simulink model "prac5"  (R2019b)
settings: Solver=VariableStepAuto  StartTime=0.0  StopTime=10  RelTol=1e-3
values from neighbouring files (symbols this model uses):
  C = 0.97    [prac5_var.m]
  Td = 0.14    [prac5_var.m]
  wn = 4.75    [prac5_var.m]
  zw2 = 2*zeta*wn    (= 0.7695)    [prac5_var.m]
undefined symbols (not defined in the file or in its folder): a1, a2, a5, a6, cputime, den, num, num1, num2
settings Model: Creator=mluser  LastModifiedBy=waltd

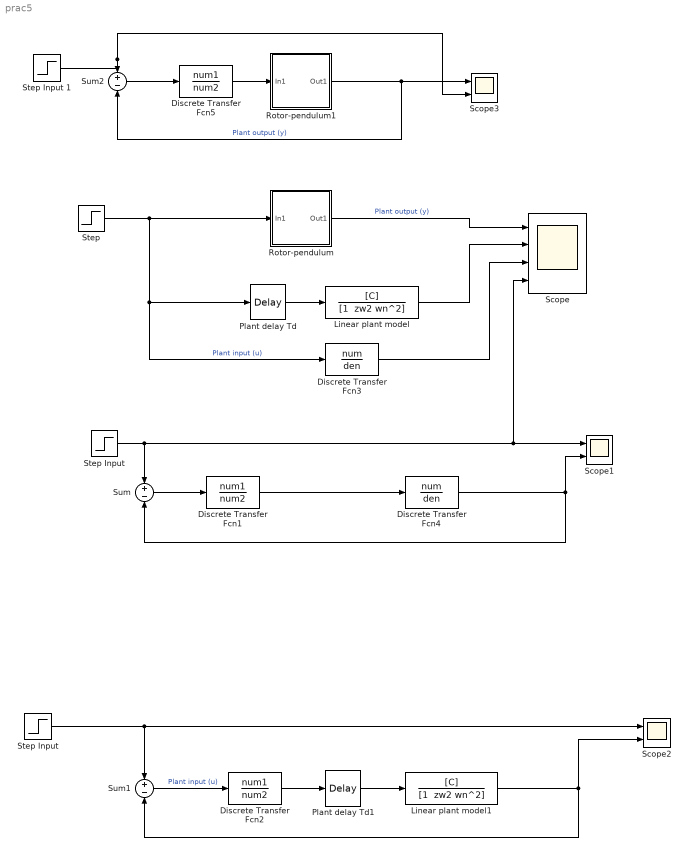
== system prac5 ==
  Discrete Transfer Fcn1 : DiscreteTransferFcn  Numerator=num1  Denominator=num2  SampleTime=0.15
  Discrete Transfer Fcn2 : DiscreteTransferFcn  Numerator=num1  Denominator=num2  SampleTime=0.15
  Discrete Transfer Fcn3 : DiscreteTransferFcn  Numerator=num  Denominator=den  SampleTime=0.15
  Discrete Transfer Fcn4 : DiscreteTransferFcn  Numerator=num  Denominator=den  SampleTime=0.15
  Discrete Transfer Fcn5 : DiscreteTransferFcn  Numerator=num1  Denominator=num2  SampleTime=0.15
  Linear plant model : TransferFcn  Numerator=[C]  Denominator="[1  zw2 wn^2]"
  Linear plant model1 : TransferFcn  Numerator=[C]  Denominator="[1  zw2 wn^2]"
  Plant delay Td : TransportDelay  DelayTime=Td
  Plant delay Td1 : TransportDelay  DelayTime=Td
  Rotor-pendulum : Subsystem  Description=Rotor pendulum
  Rotor-pendulum1 : Subsystem  Description=Rotor pendulum
  Scope : Scope  NumInputPorts=4
  Scope1 : Scope  NumInputPorts=2
  Scope2 : Scope  NumInputPorts=2
  Scope3 : Scope  NumInputPorts=2
  Step : Step  After=10  SampleTime=0
  "Step Input " : Step  After=0.5  SampleTime=0
  Step Input 1 : Step  After=0.5  SampleTime=0
  "Step Input " : Step  After=0.5  SampleTime=0
  Sum : Sum  Inputs=+-
  Sum1 : Sum  Inputs=+-
  Sum2 : Sum  Inputs=+-
  wires:
  Step/1 -> Rotor-pendulum/1(In1), Discrete Transfer Fcn3/1, Plant delay Td/1  "Plant input (u)"
  Rotor-pendulum/1(Out1) -> Scope/1  "Plant output (y)"
  Plant delay Td/1 -> Linear plant model/1
  Linear plant model/1 -> Scope/2
  Discrete Transfer Fcn1/1 -> Discrete Transfer Fcn4/1
  "Step Input "/1 -> Scope1/1, Scope/4, Sum/1
  Sum/1 -> Discrete Transfer Fcn1/1
  Plant delay Td1/1 -> Linear plant model1/1
  Sum1/1 -> Discrete Transfer Fcn2/1  "Plant input (u)"
  Linear plant model1/1 -> Scope2/2, Sum1/2
  Discrete Transfer Fcn2/1 -> Plant delay Td1/1
  "Step Input "/1 -> Scope2/1, Sum1/1
  Discrete Transfer Fcn3/1 -> Scope/3
  Discrete Transfer Fcn4/1 -> Scope1/2, Sum/2
  Discrete Transfer Fcn5/1 -> Rotor-pendulum1/1(In1)
  Rotor-pendulum1/1(Out1) -> Sum2/2, Scope3/1  "Plant output (y)"
  Step Input 1/1 -> Scope3/2, Sum2/1
  Sum2/1 -> Discrete Transfer Fcn5/1

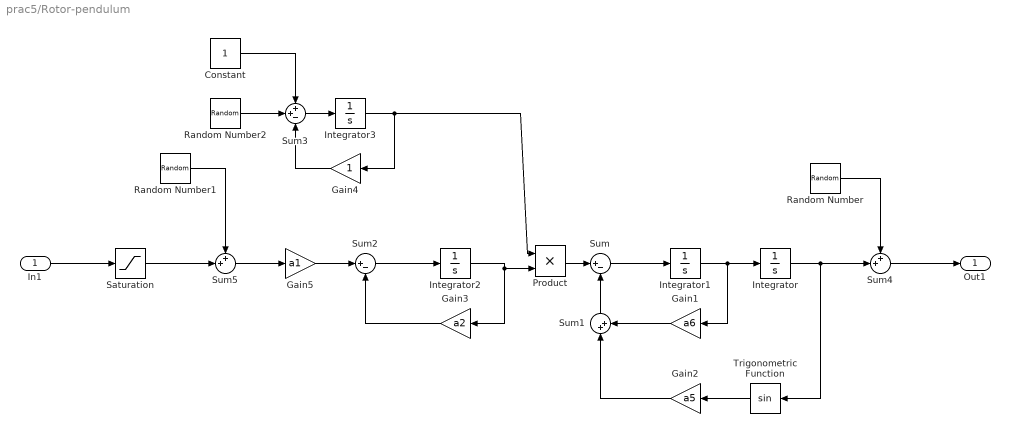
== system prac5/Rotor-pendulum ==
  In1 : Inport
  Constant : Constant
  Gain1 : Gain  Gain=a6
  Gain2 : Gain  Gain=a5
  Gain3 : Gain  Gain=a2
  Gain4 : Gain
  Gain5 : Gain  Gain=a1
  Integrator : Integrator
  Integrator1 : Integrator
  Integrator2 : Integrator
  Integrator3 : Integrator  InitialCondition=1
  Product : Product
  Random Number : RandomNumber  Variance=0.005^2  Seed=round(cputime*100)  SampleTime=0.001
  Random Number1 : RandomNumber  Variance=0.5^2  Seed=round(cputime*100)  SampleTime=0.001
  Random Number2 : RandomNumber  Variance=0.5^2  Seed=round(cputime*100)  SampleTime=0.001
  Saturation : Saturate  UpperLimit=15  LowerLimit=-15
  Sum : Sum  Inputs=|+-
  Sum1 : Sum  Inputs=|++
  Sum2 : Sum  Inputs=|+-
  Sum3 : Sum  Inputs=++-
  Sum4 : Sum  Inputs=++|
  Sum5 : Sum  Inputs=++|
  Trigonometric Function : Trigonometry
  Out1 : Outport
  wires:
  Gain2/1 -> Sum1/1
  Integrator1/1 -> Gain1/1, Integrator/1
  Sum1/1 -> Sum/2
  Gain5/1 -> Sum2/1
  Random Number1/1 -> Sum5/1
  Sum/1 -> Integrator1/1
  Sum2/1 -> Integrator2/1
  Sum5/1 -> Gain5/1
  Integrator2/1 -> Product/2, Gain3/1
  Sum4/1 -> Out1/1
  Gain1/1 -> Sum1/2
  Integrator/1 -> Sum4/2, Trigonometric Function/1
  Random Number/1 -> Sum4/1
  Trigonometric Function/1 -> Gain2/1
  Gain3/1 -> Sum2/2
  In1/1 -> Saturation/1
  Saturation/1 -> Sum5/2
  Sum3/1 -> Integrator3/1
  Product/1 -> Sum/1
  Integrator3/1 -> Gain4/1, Product/1
  Random Number2/1 -> Sum3/2
  Gain4/1 -> Sum3/3
  Constant/1 -> Sum3/1

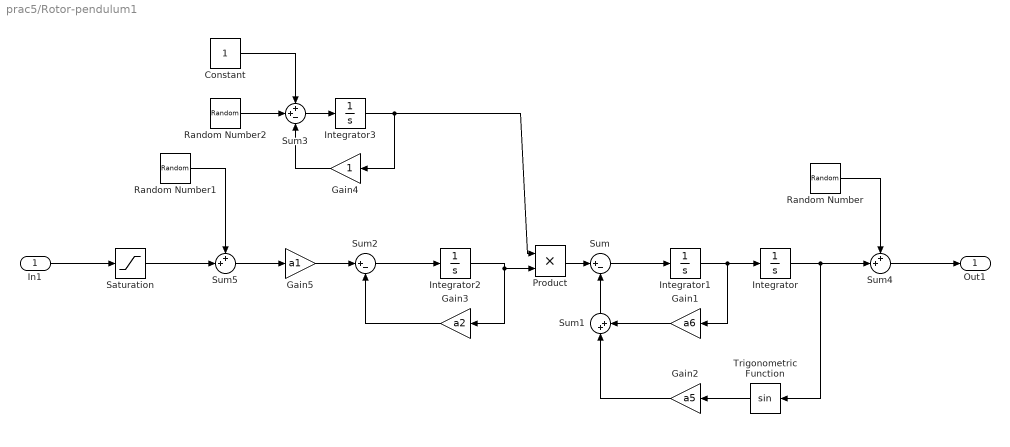
== system prac5/Rotor-pendulum1 ==
  In1 : Inport
  Constant : Constant
  Gain1 : Gain  Gain=a6
  Gain2 : Gain  Gain=a5
  Gain3 : Gain  Gain=a2
  Gain4 : Gain
  Gain5 : Gain  Gain=a1
  Integrator : Integrator
  Integrator1 : Integrator
  Integrator2 : Integrator
  Integrator3 : Integrator  InitialCondition=1
  Product : Product
  Random Number : RandomNumber  Variance=0.005^2  Seed=round(cputime*100)  SampleTime=0.001
  Random Number1 : RandomNumber  Variance=0.5^2  Seed=round(cputime*100)  SampleTime=0.001
  Random Number2 : RandomNumber  Variance=0.5^2  Seed=round(cputime*100)  SampleTime=0.001
  Saturation : Saturate  UpperLimit=15  LowerLimit=-15
  Sum : Sum  Inputs=|+-
  Sum1 : Sum  Inputs=|++
  Sum2 : Sum  Inputs=|+-
  Sum3 : Sum  Inputs=++-
  Sum4 : Sum  Inputs=++|
  Sum5 : Sum  Inputs=++|
  Trigonometric Function : Trigonometry
  Out1 : Outport
  wires:
  Gain2/1 -> Sum1/1
  Integrator1/1 -> Gain1/1, Integrator/1
  Sum1/1 -> Sum/2
  Gain5/1 -> Sum2/1
  Random Number1/1 -> Sum5/1
  Sum/1 -> Integrator1/1
  Sum2/1 -> Integrator2/1
  Sum5/1 -> Gain5/1
  Integrator2/1 -> Product/2, Gain3/1
  Sum4/1 -> Out1/1
  Gain1/1 -> Sum1/2
  Integrator/1 -> Sum4/2, Trigonometric Function/1
  Random Number/1 -> Sum4/1
  Trigonometric Function/1 -> Gain2/1
  Gain3/1 -> Sum2/2
  In1/1 -> Saturation/1
  Saturation/1 -> Sum5/2
  Sum3/1 -> Integrator3/1
  Product/1 -> Sum/1
  Integrator3/1 -> Gain4/1, Product/1
  Random Number2/1 -> Sum3/2
  Gain4/1 -> Sum3/3
  Constant/1 -> Sum3/1
